simulink model "MFWF_harness"  (R2025b)
settings: Solver=ode5  StartTime=0  StopTime=100  FixedStep=0.001  RelTol=1e-3  EnableMultiTasking=on
PreLoadFcn:
  | UIuserInputs;
model workspace (MAT data in the model file):
  t_controller = 0.01
libraries: simulink x7
settings Model: DataDictionary=topLevel.sldd  ModifiedByFormat=The MathWorks Inc.  Creator=The MathWorks, Inc.  LastModifiedBy=The MathWorks Inc.
settings SolverCC: ZeroCrossAlgorithm=Adaptive  AlgebraicLoopSolver=TrustRegion
settings DataIOCC: LimitDataPoints=on  SaveFormat=StructureWithTime  SaveOutput=off  SaveTime=off  ReturnWorkspaceOutputs=off
settings OptimizationCC: BlockReduction=off  BufferReuse=off  ExpressionDepthLimit=2147483647.0  LifeSpan=1
settings DebuggingCC: AlgebraicLoopMsg=none  UnderspecifiedInitializationDetection=Classic  MergeDetectMultiDrivingBlocksExec=none  IgnoredZcDiagnostic=none  FcnCallInpInsideContextMsg=warning  StateNameClashWarn=warning  SFUnexpectedBacktrackingDiag=warning  SFNoUnconditionalDefaultTransitionDiag=warning  SFExecutionAtInitializationDiag=none  ArithmeticOperatorsInVariantConditions=warning
settings HardwareCC: ProdBitPerPointer=32.0  ProdBitPerSizeT=32.0  ProdBitPerPtrDiffT=32.0  ProdLargestAtomicFloat=None  ProdIntDivRoundTo=Undefined  ProdEndianess=Unspecified  ProdWordSize=32.0  ProdHWDeviceType=32-bit Generic
settings ModelReferenceCC: EnableRefExpFcnMdlSchedulingChecks=on  PropagateSignalLabelsOutOfModel=off
settings SFSimCC: SimUseLocalCustomCode=off  CustomCodeUndefinedFunction=UseInterfaceOnly
settings RTWCC: RTWUseLocalCustomCode=off  GPUComputeCapability=3.5  DLArmComputeVersion=19.05
settings CodeAppCC: StateflowObjectComments=on
settings GRTTargetCC: TargetLangStandard=C89/C90 (ANSI)  CombineOutputUpdateFcns=off  GRTInterface=on
settings ConfigComp: CovMetricSettings=dw  CovSaveCumulativeToWorkspaceVar=on  CovSaveSingleToWorkspaceVar=on  CovExternalEMLEnable=off  CovSFcnEnable=off
settings SimscapeCC: SimscapeLogDataHistory=5000  SimscapeLogDecimation=1

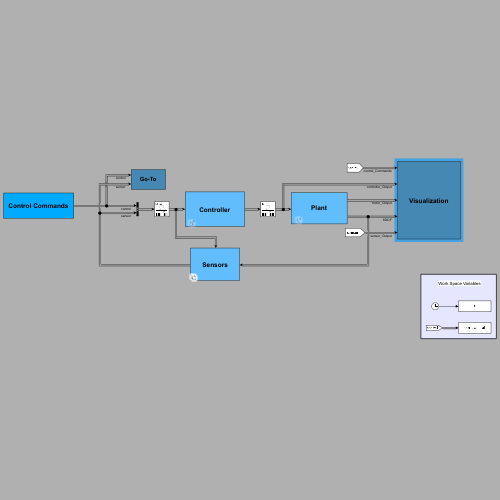
[thumbnail: Simulink's stored preview of the top-level diagram]
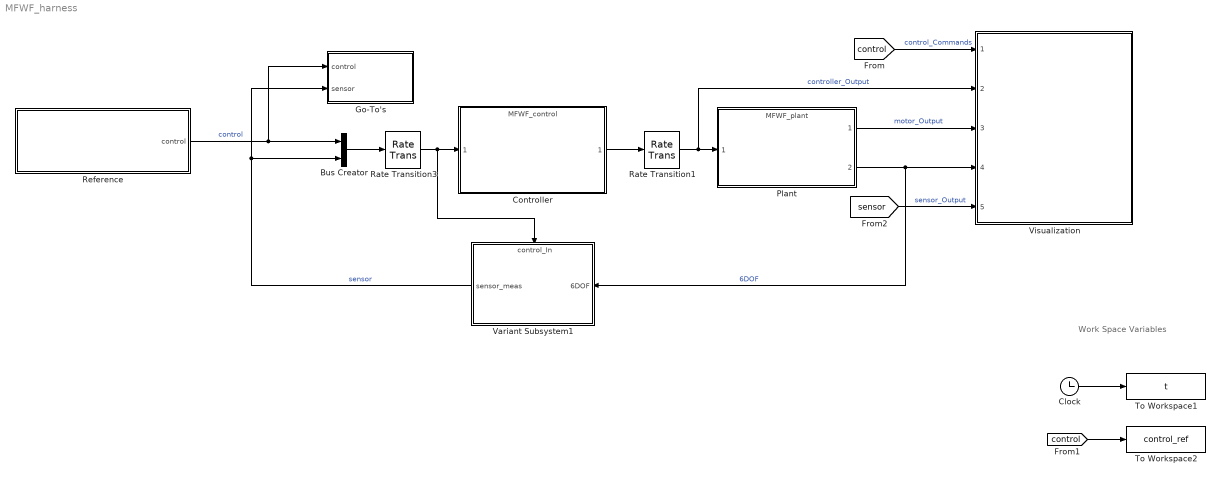
== system MFWF_harness ==
  note: Work Space Variables
  Bus Creator : BusCreator  Inputs=2
  Clock : Clock
  Controller : ModelReference  ModelNameDialog=MFWF_control  SimulationMode=Normal  ModelReferenceVersion=18.52
      mask Display: disp('Controller');
  Go-To's : Subsystem
      mask Display: disp('Go-To');
  Plant : ModelReference  ModelNameDialog=MFWF_plant  SimulationMode=Normal  ModelReferenceVersion=20.14
      mask Display: disp('Plant');
  Rate Transition1 : RateTransition
  Rate Transition3 : RateTransition
  Reference : Subsystem
      mask Display: disp('Control Commands');
  To Workspace1 : ToWorkspace  VariableName=t  SampleTime=-1
  To Workspace2 : ToWorkspace  VariableName=control_ref  SampleTime=-1
  Variant Subsystem1 : Subsystem  Variant=on
      settings: PortSchema="{\"entries\":[{\"content\":{\"sides\":[{\"content\":{\"connectorIds\":[\"In1\"]},\"type\":\"ConnectorPlacement.EquallySpacedRectSide\",\"uuid\":\"2a53bf7a-898d-4f9b-8290-2e21622b238e\"},{\"content\":{\"connectorIds\":[\"Out1\"],\"side\":\"RIGHT\"},\"type\":\"ConnectorPlacement.EquallySpacedRectSide\",\"uuid\":\"d7939d72-4210-415b-bb08-9ae3d16bbd7f\"},{\"content\":{\"connectorIds\":[\"In2\"],\"side\":\"TOP\"},\"type\":\"ConnectorPlacement.EquallySpacedRectSide\",\"uuid\":\"45ca2347-8f68-44a9-a93e-a0775ad8e94d\"}]},\"type\":\"ConnectorPlacement.EquallySpacedConnector\",\"uuid\":\"8765b8f3-4196-4bbd-8f0c-41159da5df24\"}],\"packageUris\":[\"http://schema.mathworks.com/mf0/Connector/R2020b\"],\"version\":\"1.0\"}"
      mask Display: disp('Sensors');
  Visualization : Subsystem  Description=|  ReferencedSubsystem=Visualization
      | Visualization of MFWF flight such as flyer flight path, controller output, and sensor output. Includes scope blocks in one consolidated place for viewing. Also includes 3D animation.
      | 
      | Note: 3D animation slows simulation considerably so only keep commented out when not in use).
  wires:
  [sensor] -> Visualization/5  "sensor_Output"
  [control] -> To Workspace2/1
  [control] -> Visualization/1  "control_Commands"
  Reference/1(control) -> Go-To's/1(control), Bus Creator/1  "control"
  Plant/1 -> Visualization/3  "motor_Output"
  Controller/1 -> Rate Transition1/1
  Rate Transition1/1 -> Visualization/2, Plant/1  "controller_Output"
  Rate Transition3/1 -> Variant Subsystem1/2(control_In), Controller/1
  Bus Creator/1 -> Rate Transition3/1
  Variant Subsystem1/1(sensor_meas) -> Go-To's/2(sensor), Bus Creator/2  "sensor"
  Clock/1 -> To Workspace1/1
  Plant/2 -> Variant Subsystem1/1(6DOF), Visualization/4  "6DOF"

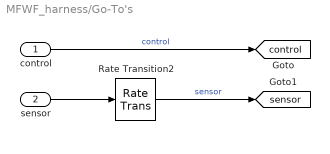
== system MFWF_harness/Go-To's ==
  control : Inport
  sensor : Inport  Port=2
  Rate Transition2 : RateTransition
  tag scope: control=global, sensor=global
  wires:
  Rate Transition2/1 -> [sensor]  "sensor"
  control/1 -> [control]  "control"
  sensor/1 -> Rate Transition2/1

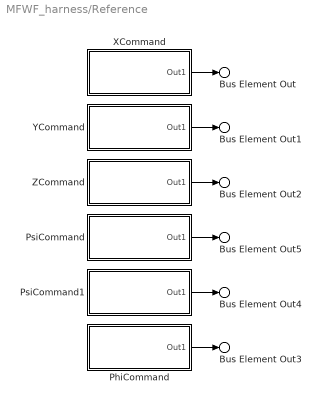
== system MFWF_harness/Reference ==
  PhiCommand : Subsystem  Variant=on
      mask Display: disp('Phi Command');
  PsiCommand : Subsystem  Variant=on
      mask Display: disp('Psi Command');
  PsiCommand1 : Subsystem  Variant=on
      mask Display: disp('Theta Command');
  XCommand : Subsystem  Variant=on
      mask Display: disp('X Command');
  YCommand : Subsystem  Variant=on
      mask Display: disp('Y Command');
  ZCommand : Subsystem  Variant=on
      mask Display: disp('Z Command');
  Bus Element Out : Outport  PortName=control  Element=x
  Bus Element Out1 : Outport  PortName=control  Element=y
  Bus Element Out2 : Outport  PortName=control  Element=z
  Bus Element Out3 : Outport  PortName=control  Element=phi
  Bus Element Out4 : Outport  PortName=control  Element=theta
  Bus Element Out5 : Outport  PortName=control  Element=psi
  wires:
  XCommand/1(Out1) -> Bus Element Out/1
  PhiCommand/1(Out1) -> Bus Element Out3/1
  PsiCommand/1(Out1) -> Bus Element Out5/1
  PsiCommand1/1(Out1) -> Bus Element Out4/1
  YCommand/1(Out1) -> Bus Element Out1/1
  ZCommand/1(Out1) -> Bus Element Out2/1

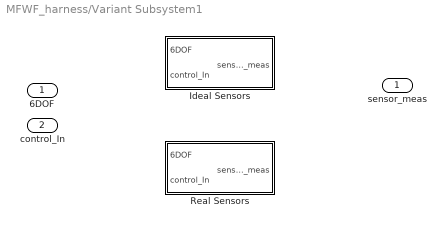
== system MFWF_harness/Variant Subsystem1 ==
  6DOF : Inport
  control_In : Inport  Port=2
  Ideal Sensors : Subsystem  VariantControl=inputs.Sensor.Ideal == 1
      mask Display: disp('Ideal Sensors');
  Real Sensors : Subsystem  VariantControl=inputs.Sensor.Ideal == 0
      mask Display: disp('Real Sensors');
  sensor_meas : Outport  OutDataTypeStr=Bus: sensor_out

== system MFWF_harness/Reference/PhiCommand ==
  Command Disabled : Subsystem  VariantControl="inputs.Commands.phiCommandEnable  == 0"
      mask Display: disp('Command Disabled');
  Command Enabled : Subsystem  VariantControl="inputs.Commands.phiCommandEnable   == 1"
      mask Display: disp('Command Enabled');
  Out1 : Outport

== system MFWF_harness/Reference/PsiCommand ==
  Command Disabled : Subsystem  VariantControl="inputs.Commands.psiCommandEnable  == 0"
      mask Display: disp('Command Disabled');
  Command Enabled : Subsystem  VariantControl="inputs.Commands.psiCommandEnable   == 1"
      mask Display: disp('Command Enabled');
  Out1 : Outport

== system MFWF_harness/Reference/PsiCommand1 ==
  Command Disabled : Subsystem  VariantControl="inputs.Commands.thetaCommandEnable  == 0"
      mask Display: disp('Command Disabled');
  Command Enabled : Subsystem  VariantControl="inputs.Commands.thetaCommandEnable   == 1"
      mask Display: disp('Command Enabled');
  Out1 : Outport

== system MFWF_harness/Reference/XCommand ==
  Command Disabled : Subsystem  VariantControl="inputs.Commands.xCommandEnable  == 0"
      mask Display: disp('Command Disabled');
  Command Enabled : Subsystem  VariantControl="inputs.Commands.xCommandEnable   == 1"
      mask Display: disp('Command Enabled');
  Out1 : Outport

== system MFWF_harness/Reference/YCommand ==
  Command Disabled : Subsystem  VariantControl="inputs.Commands.yCommandEnable  == 0"
      mask Display: disp('Command Disabled');
  Command Enabled : Subsystem  VariantControl="inputs.Commands.yCommandEnable   == 1"
      mask Display: disp('Command Enabled');
  Out1 : Outport

== system MFWF_harness/Reference/ZCommand ==
  Command Disabled : Subsystem  VariantControl="inputs.Commands.zCommandEnable  == 0"
      mask Display: disp('Command Disabled');
  Command Enabled : Subsystem  VariantControl="inputs.Commands.zCommandEnable   == 1"
      mask Display: disp('Command Enabled');
  Out1 : Outport

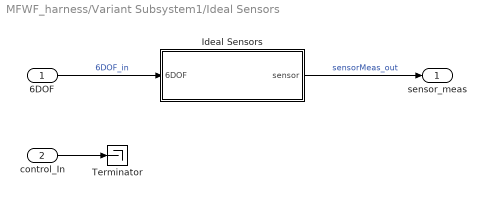
== system MFWF_harness/Variant Subsystem1/Ideal Sensors ==
  6DOF : Inport
  control_In : Inport  Port=2
  Ideal Sensors : Subsystem
      mask Display: disp('Ideal Sensors');
  Terminator : Terminator
  sensor_meas : Outport
  wires:
  6DOF/1 -> Ideal Sensors/1(6DOF)  "6DOF_in"
  Ideal Sensors/1(sensor) -> sensor_meas/1  "sensorMeas_out"
  control_In/1 -> Terminator/1

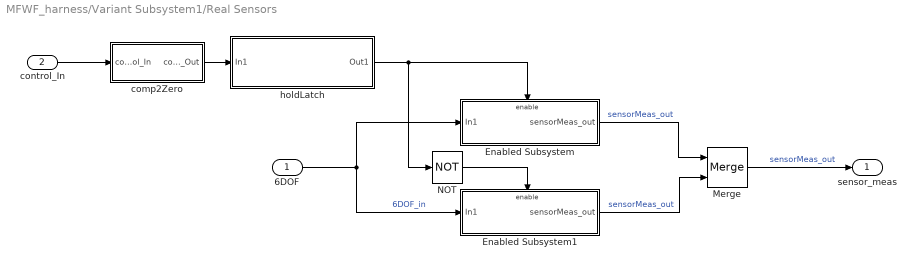
== system MFWF_harness/Variant Subsystem1/Real Sensors ==
  6DOF : Inport
  control_In : Inport  Port=2
  Enabled Subsystem : Subsystem  TreatAsAtomicUnit=on
      mask Display: disp('Real Sensor Enabled');
  Enabled Subsystem1 : Subsystem  TreatAsAtomicUnit=on
      mask Display: disp('DoF Passthrough Enabled');
  Merge : Merge
  NOT : Logic  Operator=NOT  IconShape=distinctive  AllPortsSameDT=off  OutDataTypeStr=boolean
  comp2Zero : Subsystem
      mask Display: disp("comp2Zero");
  holdLatch : Subsystem
      mask Display: disp("holdLatch");
  sensor_meas : Outport  OutDataTypeStr=Bus: sensor_out
  wires:
  6DOF/1 -> Enabled Subsystem1/1(In1), Enabled Subsystem/1(In1)  "6DOF_in"
  control_In/1 -> comp2Zero/1(control_In)
  comp2Zero/1(control_Out) -> holdLatch/1(In1)
  Enabled Subsystem/1(sensorMeas_out) -> Merge/1  "sensorMeas_out"
  Merge/1 -> sensor_meas/1  "sensorMeas_out"
  NOT/1 -> Enabled Subsystem1/Enable
  Enabled Subsystem1/1(sensorMeas_out) -> Merge/2  "sensorMeas_out"
  holdLatch/1(Out1) -> Enabled Subsystem/Enable, NOT/1

== system MFWF_harness/Reference/PhiCommand/Command Disabled ==
  Ground : Ground
  Out1 : Outport
  wires:
  Ground/1 -> Out1/1

== system MFWF_harness/Reference/PhiCommand/Command Enabled ==
  From Workspace : FromWorkspace  VariableName=inputs.Commands.phiCommand  Interpolate=off  OutputAfterFinalValue=Setting to zero
  Out1 : Outport
  wires:
  From Workspace/1 -> Out1/1

== system MFWF_harness/Reference/PsiCommand/Command Disabled ==
  Ground : Ground
  Out1 : Outport
  wires:
  Ground/1 -> Out1/1

== system MFWF_harness/Reference/PsiCommand/Command Enabled ==
  From Workspace : FromWorkspace  VariableName=inputs.Commands.psiCommand  Interpolate=off  OutputAfterFinalValue=Setting to zero
  Out1 : Outport
  wires:
  From Workspace/1 -> Out1/1

== system MFWF_harness/Reference/PsiCommand1/Command Disabled ==
  Ground : Ground
  Out1 : Outport
  wires:
  Ground/1 -> Out1/1

== system MFWF_harness/Reference/PsiCommand1/Command Enabled ==
  From Workspace : FromWorkspace  VariableName=inputs.Commands.thetaCommand  Interpolate=off  OutputAfterFinalValue=Setting to zero
  Out1 : Outport
  wires:
  From Workspace/1 -> Out1/1

== system MFWF_harness/Reference/XCommand/Command Disabled ==
  Ground : Ground
  Out1 : Outport
  wires:
  Ground/1 -> Out1/1

== system MFWF_harness/Reference/XCommand/Command Enabled ==
  From Workspace : FromWorkspace  VariableName=inputs.Commands.xCommand  Interpolate=off  OutputAfterFinalValue=Setting to zero
  Out1 : Outport
  wires:
  From Workspace/1 -> Out1/1

== system MFWF_harness/Reference/YCommand/Command Disabled ==
  Ground : Ground
  Out1 : Outport
  wires:
  Ground/1 -> Out1/1

== system MFWF_harness/Reference/YCommand/Command Enabled ==
  From Workspace1 : FromWorkspace  VariableName=inputs.Commands.yCommand  Interpolate=off  OutputAfterFinalValue=Setting to zero
  Out1 : Outport
  wires:
  From Workspace1/1 -> Out1/1

== system MFWF_harness/Reference/ZCommand/Command Disabled ==
  Ground : Ground
  Out1 : Outport
  wires:
  Ground/1 -> Out1/1

== system MFWF_harness/Reference/ZCommand/Command Enabled ==
  From Workspace : FromWorkspace  VariableName=inputs.Commands.zCommand  Interpolate=off  OutputAfterFinalValue=Setting to zero
  Out1 : Outport
  wires:
  From Workspace/1 -> Out1/1

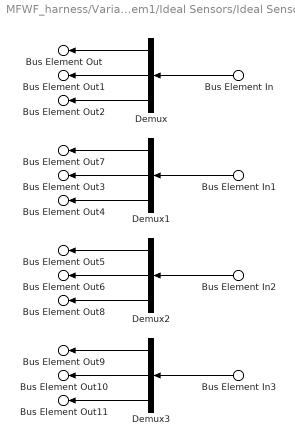
== system MFWF_harness/Variant Subsystem1/Ideal Sensors/Ideal Sensors ==
  Bus Element In : Inport  PortName=6DOF  Element=inertial.position
  Bus Element In3 : Inport  PortName=6DOF  Element=inertial.velocity
  Bus Element In1 : Inport  PortName=6DOF  Element=body.angles
  Bus Element In2 : Inport  PortName=6DOF  Element=body.angularRate
  Demux{,1..3} (4 alike) : Demux  Outputs=3
  Bus Element Out : Outport  PortName=sensor  Element=x
  Bus Element Out1 : Outport  PortName=sensor  Element=y
  Bus Element Out7 : Outport  PortName=sensor  Element=phi
  Bus Element Out3 : Outport  PortName=sensor  Element=theta
  Bus Element Out4 : Outport  PortName=sensor  Element=psi
  Bus Element Out5 : Outport  PortName=sensor  Element=p
  Bus Element Out6 : Outport  PortName=sensor  Element=q
  Bus Element Out8 : Outport  PortName=sensor  Element=r
  Bus Element Out9 : Outport  PortName=sensor  Element=Vx
  Bus Element Out10 : Outport  PortName=sensor  Element=Vy
  Bus Element Out11 : Outport  PortName=sensor  Element=Vz
  Bus Element Out2 : Outport  PortName=sensor  Element=z
  wires:
  Demux1/1 -> Bus Element Out7/1
  Demux2/3 -> Bus Element Out8/1
  Demux1/3 -> Bus Element Out4/1
  Demux3/2 -> Bus Element Out10/1
  Demux1/2 -> Bus Element Out3/1
  Bus Element In1/1 -> Demux1/1
  Demux/2 -> Bus Element Out1/1
  Demux/1 -> Bus Element Out/1
  Demux3/1 -> Bus Element Out9/1
  Bus Element In2/1 -> Demux2/1
  Demux3/3 -> Bus Element Out11/1
  Bus Element In/1 -> Demux/1
  Demux/3 -> Bus Element Out2/1
  Demux2/2 -> Bus Element Out6/1
  Demux2/1 -> Bus Element Out5/1
  Bus Element In3/1 -> Demux3/1

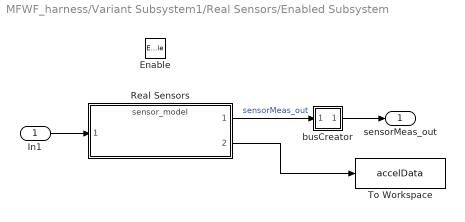
== system MFWF_harness/Variant Subsystem1/Real Sensors/Enabled Subsystem ==
  In1 : Inport
  Enable : EnablePort
  Real Sensors : ModelReference  Description=The sensor model simulates the installed sensors on the MFWF and adds noise and error due to sensor limitations to the flyer's controller inputs. The sensor model is made up two main sensors, the 9DOF inertial measurement unit (IMU) and the time of flight (ToF) sensor.  ModelNameDialog=sensor_model  SimulationMode=Normal  ModelReferenceVersion=8.58
      mask Display: disp('Real Sensors');
  To Workspace : ToWorkspace  VariableName=accelData  SampleTime=-1
  busCreator : Subsystem
  sensorMeas_out : Outport  OutDataTypeStr=Bus: sensor_out
  wires:
  In1/1 -> Real Sensors/1
  busCreator/1(sensorMeas_out) -> sensorMeas_out/1
  Real Sensors/1 -> busCreator/1(sensorMeas_in)  "sensorMeas_out"
  Real Sensors/2 -> To Workspace/1

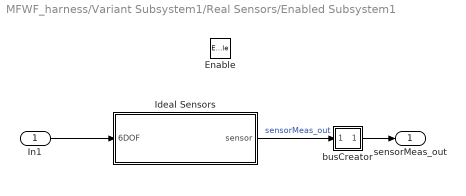
== system MFWF_harness/Variant Subsystem1/Real Sensors/Enabled Subsystem1 ==
  In1 : Inport
  Enable : EnablePort
  Ideal Sensors : Subsystem
      mask Display: disp('Ideal Sensors');
  busCreator : Subsystem
  sensorMeas_out : Outport  OutDataTypeStr=Bus: sensor_out
  wires:
  busCreator/1(sensorMeas_out) -> sensorMeas_out/1
  In1/1 -> Ideal Sensors/1(6DOF)
  Ideal Sensors/1(sensor) -> busCreator/1(sensorMeas_in)  "sensorMeas_out"

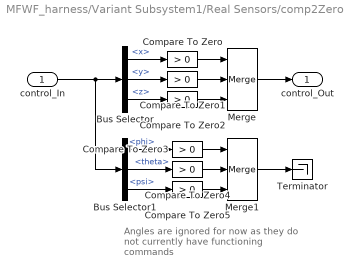
== system MFWF_harness/Variant Subsystem1/Real Sensors/comp2Zero ==
  note: Angles are ignored for now as they do not currently have functioning commands
  control_In : Inport
  Bus Selector : BusSelector  OutputSignals=control.x,control.y,control.z
  Bus Selector1 : BusSelector  OutputSignals=control.phi,control.theta,control.psi
  Compare To Zero{,1..5} (6 alike) : simulink/Logic and Bit Operations/Compare To Zero  relop=>  OutDataTypeStr=boolean
  Merge : Merge  Inputs=3
  Merge1 : Merge  Inputs=3
  Terminator : Terminator
  control_Out : Outport
  wires:
  Bus Selector/1 -> Compare To Zero/1  "<x>"
  Bus Selector/3 -> Compare To Zero2/1  "<z>"
  Bus Selector/2 -> Compare To Zero1/1  "<y>"
  Compare To Zero1/1 -> Merge/2
  Compare To Zero2/1 -> Merge/3
  Compare To Zero/1 -> Merge/1
  control_In/1 -> Bus Selector1/1, Bus Selector/1
  Compare To Zero5/1 -> Merge1/3
  Compare To Zero4/1 -> Merge1/2
  Compare To Zero3/1 -> Merge1/1
  Bus Selector1/2 -> Compare To Zero4/1  "<theta>"
  Bus Selector1/3 -> Compare To Zero5/1  "<psi>"
  Bus Selector1/1 -> Compare To Zero3/1  "<phi>"
  Merge1/1 -> Terminator/1
  Merge/1 -> control_Out/1

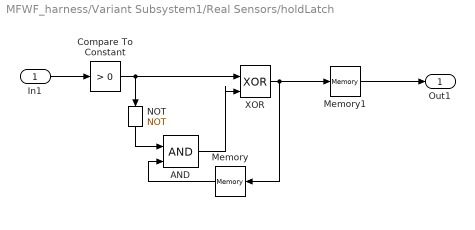
== system MFWF_harness/Variant Subsystem1/Real Sensors/holdLatch ==
  In1 : Inport
  AND : Logic  IconShape=distinctive  AllPortsSameDT=off  OutDataTypeStr=boolean
  Compare To Constant : simulink/Logic and Bit Operations/Compare To Constant  relop=>  const=0  OutDataTypeStr=boolean
  Memory : Memory
  Memory1 : Memory
  NOT : Logic  Operator=NOT  IconShape=distinctive  AllPortsSameDT=off  OutDataTypeStr=boolean
  XOR : Logic  Operator=XOR  IconShape=distinctive  AllPortsSameDT=off  OutDataTypeStr=boolean
  Out1 : Outport
  wires:
  In1/1 -> Compare To Constant/1
  XOR/1 -> Memory1/1, Memory/1
  Compare To Constant/1 -> NOT/1, XOR/1
  Memory/1 -> AND/2
  AND/1 -> XOR/2
  NOT/1 -> AND/1
  Memory1/1 -> Out1/1

== system MFWF_harness/Variant Subsystem1/Real Sensors/Enabled Subsystem/busCreator ==
  sensorMeas_in : Inport
  Bus Creator : BusCreator  Inputs=12
  Bus Selector : BusSelector  OutputSignals=x,y,psi,theta,phi,p,q,r,Vx,Vy,Vz,z
  sensorMeas_out : Outport  OutDataTypeStr=Bus: sensor_out
  wires:
  Bus Selector/12 -> Bus Creator/12  "<z>"
  Bus Selector/9 -> Bus Creator/9  "<Vx>"
  sensorMeas_in/1 -> Bus Selector/1
  Bus Selector/3 -> Bus Creator/3  "<psi>"
  Bus Selector/6 -> Bus Creator/6  "<p>"
  Bus Selector/10 -> Bus Creator/10  "<Vy>"
  Bus Selector/5 -> Bus Creator/5  "<phi>"
  Bus Selector/11 -> Bus Creator/11  "<Vz>"
  Bus Selector/7 -> Bus Creator/7  "<q>"
  Bus Selector/4 -> Bus Creator/4  "<theta>"
  Bus Selector/2 -> Bus Creator/2  "<y>"
  Bus Selector/8 -> Bus Creator/8  "<r>"
  Bus Selector/1 -> Bus Creator/1  "<x>"
  Bus Creator/1 -> sensorMeas_out/1

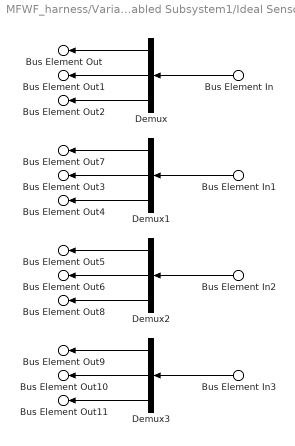
== system MFWF_harness/Variant Subsystem1/Real Sensors/Enabled Subsystem1/Ideal Sensors ==
  Bus Element In : Inport  PortName=6DOF  Element=inertial.position
  Bus Element In3 : Inport  PortName=6DOF  Element=inertial.velocity
  Bus Element In1 : Inport  PortName=6DOF  Element=body.angles
  Bus Element In2 : Inport  PortName=6DOF  Element=body.angularRate
  Demux{,1..3} (4 alike) : Demux  Outputs=3
  Bus Element Out : Outport  PortName=sensor  Element=x
  Bus Element Out1 : Outport  PortName=sensor  Element=y
  Bus Element Out7 : Outport  PortName=sensor  Element=phi
  Bus Element Out3 : Outport  PortName=sensor  Element=theta
  Bus Element Out4 : Outport  PortName=sensor  Element=psi
  Bus Element Out5 : Outport  PortName=sensor  Element=p
  Bus Element Out6 : Outport  PortName=sensor  Element=q
  Bus Element Out8 : Outport  PortName=sensor  Element=r
  Bus Element Out9 : Outport  PortName=sensor  Element=Vx
  Bus Element Out10 : Outport  PortName=sensor  Element=Vy
  Bus Element Out11 : Outport  PortName=sensor  Element=Vz
  Bus Element Out2 : Outport  PortName=sensor  Element=z
  wires:
  Demux1/1 -> Bus Element Out7/1
  Demux2/3 -> Bus Element Out8/1
  Demux1/3 -> Bus Element Out4/1
  Demux3/2 -> Bus Element Out10/1
  Demux1/2 -> Bus Element Out3/1
  Bus Element In1/1 -> Demux1/1
  Demux/2 -> Bus Element Out1/1
  Demux/1 -> Bus Element Out/1
  Demux3/1 -> Bus Element Out9/1
  Bus Element In2/1 -> Demux2/1
  Demux3/3 -> Bus Element Out11/1
  Bus Element In/1 -> Demux/1
  Demux/3 -> Bus Element Out2/1
  Demux2/2 -> Bus Element Out6/1
  Demux2/1 -> Bus Element Out5/1
  Bus Element In3/1 -> Demux3/1

== system MFWF_harness/Variant Subsystem1/Real Sensors/Enabled Subsystem1/busCreator ==
  sensorMeas_in : Inport
  Bus Creator : BusCreator  Inputs=12
  Bus Selector : BusSelector  OutputSignals=x,y,psi,theta,phi,p,q,r,Vx,Vy,Vz,z
  sensorMeas_out : Outport  OutDataTypeStr=Bus: sensor_out
  wires:
  Bus Creator/1 -> sensorMeas_out/1
  Bus Selector/1 -> Bus Creator/1  "<x>"
  Bus Selector/8 -> Bus Creator/8  "<r>"
  Bus Selector/2 -> Bus Creator/2  "<y>"
  Bus Selector/4 -> Bus Creator/4  "<theta>"
  Bus Selector/7 -> Bus Creator/7  "<q>"
  Bus Selector/11 -> Bus Creator/11  "<Vz>"
  Bus Selector/5 -> Bus Creator/5  "<phi>"
  Bus Selector/10 -> Bus Creator/10  "<Vy>"
  Bus Selector/6 -> Bus Creator/6  "<p>"
  Bus Selector/3 -> Bus Creator/3  "<psi>"
  sensorMeas_in/1 -> Bus Selector/1
  Bus Selector/9 -> Bus Creator/9  "<Vx>"
  Bus Selector/12 -> Bus Creator/12  "<z>"
